simulink model "playground"  (R2024a)
settings: Solver=ode45  StartTime=0.0  StopTime=10.0  FixedStep=0.001  RelTol=1e-3
values from neighbouring files (symbols this model uses):
  a_r = 1.14 * 10^(-7)    (= 1.14e-07)    [start.m]    (also in startEnglPaper.m = 0.033; startReduced.m)
  a_rS = b    (= 0.033)    [startEnglPaper.m]
  A_x = 0.25    [playgrounMat.m]    (also in start.m; startEnglPaper.m; startReduced.m)
  A_y = 0.25    [playgrounMat.m]    (also in start.m; startEnglPaper.m; startReduced.m)
  A_z = 0.25    [playgrounMat.m]    (also in start.m; startEnglPaper.m; startReduced.m)
  b = 1.14 * 10^(-7)    (= 1.14e-07)    [start.m]    (also in startEnglPaper.m = 0.033; startReduced.m)
  g = 9.81    [playgrounMat.m]    (also in start.m; startEnglPaper.m; startReduced.m)
  gamma_d = pi/3    (= 1.0471975512)    [start.m]    (also in startReduced.m)
  I_r = 5.38 * 10 ^ (-5)    (= 5.38e-05)    [start.m]    (also in startEnglPaper.m = 3.38e-05; startReduced.m)
  I_x = 0.0151    [start.m]    (also in startEnglPaper.m = 0.004856; startReduced.m)
  I_y = 0.253    [start.m]    (also in startEnglPaper.m = 0.004856; startReduced.m)
  I_z = 0.0151    [start.m]    (also in startEnglPaper.m = 0.008801; startReduced.m)
  IrS = 5.38 * 10^(-5)    (= 5.38e-05)    [startEnglPaper.m]
  IxS = 0.0151    [startEnglPaper.m]
  IyS = IxS    (= 0.0151)    [startEnglPaper.m]
  IzS = 0.0253    [startEnglPaper.m]
  k = 1.045 * 10^(-11)    (= 1.045e-11)    [start.m]    (also in startEnglPaper.m = 2.98e-06; startReduced.m)
  K_gamma_D1 = K(1)    [playgrounMat.m]
  K_gamma_I1 = K(3)    [playgrounMat.m]
  K_gamma_P1 = K(2)    [playgrounMat.m]
  K_phi_D1 = 0.047    [startEnglPaper.m]
  K_phi_D11 = 0.093    [startEnglPaper.m]
  K_phi_D2 = 9.6    [startEnglPaper.m]
  K_phi_D22 = 19.2    [startEnglPaper.m]
  K_phi_DS = 0.14    [startEnglPaper.m]
  K_phi_I11 = 1.27    [startEnglPaper.m]
  K_phi_I22 = 262.144    [startEnglPaper.m]
  K_phi_P1 = 0.11    [startEnglPaper.m]
  K_phi_P11 = 0.5966    [startEnglPaper.m]
  K_phi_P2 = 23.04    [startEnglPaper.m]
  K_phi_P22 = 122.88    [startEnglPaper.m]
  K_phi_PS = 0.35    [startEnglPaper.m]
  K_psi_D = 40    [start.m]    (also in startEnglPaper.m = 9.6; startReduced.m)
  K_psi_D1 = 0.0844    [startEnglPaper.m]
  K_psi_D2 = 9.6    [startEnglPaper.m]
  K_psi_D22 = 19.2    [startEnglPaper.m]
  K_psi_DS = 0.24    [startEnglPaper.m]
  K_psi_I22 = 262.144    [startEnglPaper.m]
  K_psi_P = 143    [start.m]    (also in startEnglPaper.m = 23.04; startReduced.m)
  K_psi_P1 = 0.202    [startEnglPaper.m]
  K_psi_P2 = 23.04    [startEnglPaper.m]
  K_psi_P22 = 122.88    [startEnglPaper.m]
  K_psi_PS = 0.58    [startEnglPaper.m]
  K_theta_D = 58    [start.m]    (also in startEnglPaper.m = 9.6; startReduced.m)
  K_theta_D1 = 0.047    [startEnglPaper.m]
  K_theta_D2 = 9.6    [startEnglPaper.m]
  K_theta_D22 = 19.2    [startEnglPaper.m]
  K_theta_DS = 0.14    [startEnglPaper.m]
  K_theta_I22 = 262.144    [startEnglPaper.m]
  K_theta_P = 141    [start.m]    (also in startEnglPaper.m = 23.04; startReduced.m)
  K_theta_P1 = 0.11    [startEnglPaper.m]
  K_theta_P2 = 23.04    [startEnglPaper.m]
  K_theta_P22 = 122.88    [startEnglPaper.m]
  K_theta_PS = 0.35    [startEnglPaper.m]
  K_y_D = 13.58    [start.m]    (also in startReduced.m)
  K_y_P = 33.18    [start.m]    (also in startReduced.m)
  K_z_D1 = 4.42    [startEnglPaper.m]
  K_z_D2 = 4.42/m + A_z/m    (= 9.60905349794)    [startEnglPaper.m]
  K_z_DS = 13.58    [startEnglPaper.m]
  K_z_P1 = 11.2    [startEnglPaper.m]
  K_z_P2 = 11.2/m + A_z/m    (= 23.5596707819)    [startEnglPaper.m]
  K_z_PS = 33.18    [startEnglPaper.m]
  kl = 3 * 10^(-6)    (= 3e-06)    [startEnglPaper.m]
  l = 0.225    [start.m]    (also in startEnglPaper.m; startReduced.m)
  m = 1.44    [playgrounMat.m]    (also in start.m; startEnglPaper.m = 0.486; startReduced.m)
  m_s = [1/4 0 -1/(2*l) -1/(4*a_r); 1/4 -1/(2*l) 0 1/(4*a_r); 1/4 0 1/(2*l) -1/(4*a_r); 1/4 1/(2*l) 0 1/(4*a_r)]    [start.m]    (also in startReduced.m)
  mS = 1.44    [startEnglPaper.m]
  phi_d = 0.2    [startEnglPaper.m]
  phi_DesS = 0.2    [startEnglPaper.m]
  phi_init = 0    [startEnglPaper.m]
  phi_iS = 0;   deg2rad(10)    [startEnglPaper.m]
  psi_d = pi/5    (= 0.628318530718)    [start.m]    (also in startEnglPaper.m = 0.15; startReduced.m)
  psi_DesS = 0.15    [startEnglPaper.m]
  psi_init = 0    [startEnglPaper.m]
  psi_iS = 0    [startEnglPaper.m]
  theta_d = pi/4    (= 0.785398163397)    [start.m]    (also in startEnglPaper.m = 0.3; startReduced.m)
  theta_DesS = -0.1 * -3    (= 0.3)    [startEnglPaper.m]
  theta_init = 0    [startEnglPaper.m]
  theta_iS = 0    [startEnglPaper.m]
  x_init = 0    [startEnglPaper.m]
  x_iS = 0    [startEnglPaper.m]
  y_init = 0    [startEnglPaper.m]
  y_iS = 0    [startEnglPaper.m]
  z_d = 0.05 * 0    (= 0)    [startEnglPaper.m]
  z_DesS = 0.1    [startEnglPaper.m]
  z_init = 0    [startEnglPaper.m]
  z_iS = 0.0    (= 0)    [startEnglPaper.m]
undefined symbols (not defined in the file or in its folder): m_s_my
libraries: slpidlib x14
(part 2 of 4)

== system playground/ST_constants_useIX/OMEGA_2_TAU ==
  w1 : Inport
  w2 : Inport  Port=2
  w3 : Inport  Port=3
  w4 : Inport  Port=4
  Constant : Constant  Value=kl*l
  Constant1 : Constant  Value=kl*l
  Constant11 : Constant  Value=kl
  Constant7 : Constant  Value=a_rS
  Current z : Display
  Current z1 : Display
  Gyroscope : MATLAB Function  TreatAsAtomicUnit=on
  MATLAB Function : MATLAB Function  TreatAsAtomicUnit=on
  MATLAB Function1 : MATLAB Function  TreatAsAtomicUnit=on
  MATLAB Function2 : MATLAB Function  TreatAsAtomicUnit=on
  MATLAB Function3 : MATLAB Function  TreatAsAtomicUnit=on
  wR : Outport
  T_w : Outport  Port=2
  tau_phiW : Outport  Port=3
  tau_thetaW : Outport  Port=4
  tau_psiW : Outport  Port=5
  wires:
  w1/1 -> Gyroscope/1(w_1), MATLAB Function3/1(w1), MATLAB Function2/1(w1), MATLAB Function/1(w1)
  w2/1 -> Gyroscope/2(w_2), MATLAB Function3/2(w2), MATLAB Function1/1(w2), MATLAB Function/2(w2)
  w3/1 -> Gyroscope/3(w_3), MATLAB Function3/3(w3), MATLAB Function2/2(w3), MATLAB Function/3(w3)
  w4/1 -> Gyroscope/4(w_4), MATLAB Function1/2(w4), MATLAB Function/4(w4), MATLAB Function3/4(w4)
  Constant7/1 -> MATLAB Function3/5(b)
  Constant1/1 -> MATLAB Function2/3(kl)
  Constant/1 -> MATLAB Function1/3(kl)
  Constant11/1 -> MATLAB Function/5(k)
  MATLAB Function/1(T) -> Current z/1, T_w/1
  MATLAB Function1/1(tau_phi) -> Current z1/1, tau_phiW/1
  MATLAB Function2/1(tau_theta) -> tau_thetaW/1
  MATLAB Function3/1(tau_psi) -> tau_psiW/1
  Gyroscope/1(w_Gamma) -> wR/1

== system playground/ST_constants_useIX/Omega SAT ==
  w1 : Inport
  w2 : Inport  Port=2
  w3 : Inport  Port=3
  w4 : Inport  Port=4
  Current z{1..4} (4 alike) : Display
  Gain{1..4} (4 alike) : Gain  Gain=2*pi/60
  Manual Switch1 : ManualSwitch
  Manual Switch3 : ManualSwitch
  Manual Switch4 : ManualSwitch
  Manual Switch5 : ManualSwitch  CurrentSetting=0
  Sat w1 : Saturate  UpperLimit=13000  LowerLimit=1000
  Sat w2 : Saturate  UpperLimit=12500  LowerLimit=1000
  Sat w3 : Saturate  UpperLimit=12500  LowerLimit=1000
  Sat w4 : Saturate  UpperLimit=11500  LowerLimit=1000
  оборотов/мин{1..4} (4 alike) : Gain  Gain=60/(2*pi)
  w1S : Outport
  w2S : Outport  Port=2
  w3S : Outport  Port=3
  w4S : Outport  Port=4
  wires:
  w1/1 -> оборотов/мин1/1
  Gain3/1 -> Current z1/1, w3S/1  "рад/сек"
  Gain1/1 -> Current z3/1, w1S/1  "рад/сек"
  Gain2/1 -> Current z2/1, w2S/1  "рад/сек"
  Gain4/1 -> Current z4/1, w4S/1  "рад/сек"
  оборотов/мин1/1 -> Sat w1/1, Manual Switch1/1  "w1"
  Sat w1/1 -> Manual Switch1/2
  Manual Switch1/1 -> Gain1/1
  оборотов/мин2/1 -> Manual Switch3/1, Sat w2/1  "w2"
  w2/1 -> оборотов/мин2/1
  Sat w2/1 -> Manual Switch3/2
  Manual Switch3/1 -> Gain2/1
  оборотов/мин3/1 -> Sat w3/1, Manual Switch4/1  "w3"
  w3/1 -> оборотов/мин3/1
  Sat w3/1 -> Manual Switch4/2
  Manual Switch4/1 -> Gain3/1
  оборотов/мин4/1 -> Sat w4/1, Manual Switch5/1  "w4"
  w4/1 -> оборотов/мин4/1
  Sat w4/1 -> Manual Switch5/2
  Manual Switch5/1 -> Gain4/1

== system playground/ST_constants_useIX/TAU_2_OMEGA ==
  T : Inport
  tau_phi : Inport  Port=2
  tau_theta : Inport  Port=3
  tau_psi : Inport  Port=4
  Constant11 : Constant  Value=kl
  Constant12 : Constant  Value=l
  Constant7 : Constant  Value=a_rS
  Current z{,1..7} (8 alike) : Display
  MATLAB Function1 : MATLAB Function  TreatAsAtomicUnit=on
  Scope : Scope
  Sqrt{1..4} (4 alike) : Sqrt
  w1 : Outport
  w2 : Outport  Port=2
  w3 : Outport  Port=3
  w4 : Outport  Port=4
  wires:
  Constant11/1 -> MATLAB Function1/5(k)
  Constant12/1 -> MATLAB Function1/6(l)
  Constant7/1 -> MATLAB Function1/7(b)
  T/1 -> Current z4/1, MATLAB Function1/1(T)
  tau_phi/1 -> Current z5/1, MATLAB Function1/2(tau_phi)
  tau_theta/1 -> MATLAB Function1/3(tau_theta)
  tau_psi/1 -> Scope/1, Current z6/1, MATLAB Function1/4(tau_psi)
  Sqrt1/1 -> Current z/1, w1/1  "рад/сек"
  Sqrt2/1 -> Current z3/1, w2/1  "рад/сек"
  Sqrt3/1 -> Current z2/1, w3/1  "рад/сек"
  Sqrt4/1 -> Current z1/1, w4/1  "рад/сек"
  MATLAB Function1/1(omega_1) -> Sqrt1/1
  MATLAB Function1/2(omega_2) -> Current z7/1, Sqrt2/1
  MATLAB Function1/3(omega_3) -> Sqrt3/1
  MATLAB Function1/4(omega_4) -> Sqrt4/1

== system playground/ST_constants_useIX/XYZ POSITION ==
  T : Inport
  phi : Inport  Port=2
  theta : Inport  Port=3
  psi : Inport  Port=4
  Constant : Constant  Value=mS
  Constant1 : Constant  Value=A_x
  Constant2 : Constant  Value=A_y
  Constant3 : Constant  Value=A_z
  Integrator4 : Integrator
  XYZ : MATLAB Function  TreatAsAtomicUnit=on
  integrator1 : Integrator
  integrator2 : Integrator
  xinit : Integrator  InitialCondition=x_iS
  yinit : Integrator  InitialCondition=y_iS
  zinit : Integrator  InitialCondition=z_iS
  x : Outport
  y : Outport  Port=2
  z : Outport  Port=3
  wires:
  Constant3/1 -> XYZ/5(Az)
  Constant2/1 -> XYZ/4(Ay)
  integrator1/1 -> [dx], xinit/1
  integrator2/1 -> [dy], yinit/1
  Integrator4/1 -> [dz], zinit/1
  XYZ/2(ddy) -> integrator2/1
  XYZ/1(ddx) -> integrator1/1
  XYZ/3(ddz) -> Integrator4/1
  Constant1/1 -> XYZ/3(Ax)
  Constant/1 -> XYZ/2(m)
  T/1 -> XYZ/1(T)
  phi/1 -> XYZ/6(phi)
  theta/1 -> XYZ/7(theta)
  psi/1 -> XYZ/8(psi)
  [dx] -> XYZ/9(dx)
  [dy] -> XYZ/10(dy)
  [dz] -> XYZ/11(dz)
  xinit/1 -> x/1
  yinit/1 -> y/1
  zinit/1 -> z/1

== system playground/quad_PID_Simpl/9_form_omega ==
  tau_gamma : Inport
  tau_theta : Inport  Port=2
  tau_psi : Inport  Port=3
  omega_r : Inport  Port=4
  Constant1 : Constant  Value=I_z
  Constant10 : Constant  Value=I_r
  Constant11 : Constant  Value=I_y
  Constant12 : Constant  Value=I_x
  Constant2 : Constant  Value=I_z
  Constant3 : Constant  Value=I_r
  Constant4 : Constant  Value=I_y
  Constant5 : Constant  Value=I_x
  Constant6 : Constant  Value=I_y
  Constant7 : Constant  Value=I_z
  Constant8 : Constant  Value=I_x
  Integrator1 : Integrator
  Integrator2 : Integrator
  Integrator3 : Integrator
  omega_r1 : InportShadow  Port=4
  omega_x' : MATLAB Function  TreatAsAtomicUnit=on
  omega_y' : MATLAB Function  TreatAsAtomicUnit=on
  omega_z' : MATLAB Function  TreatAsAtomicUnit=on
  omega_x : Outport
  omega_y : Outport  Port=2
  omega_z : Outport  Port=3
  wires:
  Constant11/1 -> omega_y'/3(I_y)  "I_y"
  Constant12/1 -> omega_y'/2(I_x)  "I_x"
  Constant7/1 -> omega_y'/1(I_z)  "I_y"
  Constant3/1 -> omega_z'/4(I_r)  "I_r"
  Constant2/1 -> omega_z'/3(I_z)  "I_y"
  Constant5/1 -> omega_z'/2(I_x)  "I_x"
  Constant4/1 -> omega_z'/1(I_y)  "I_y"
  omega_r1/1 -> omega_x'/7(omega_r)  "omega_r"
  Constant1/1 -> omega_x'/3(I_z)  "I_y"
  omega_r/1 -> omega_z'/7(omega_r)  "omega_r"
  tau_theta/1 -> omega_z'/8(tau_theta)  "tau_theta"
  tau_psi/1 -> omega_y'/6(tau_psi)  "tau_psi"
  Integrator1/1 -> omega_y/1, omega_x'/5(omega_y), omega_z'/5(omega_y)  "omega_y"
  Integrator2/1 -> omega_z/1, omega_y'/5(omega_z), omega_x'/6(omega_z)  "omega_z"
  omega_z'/1(domega_z) -> Integrator2/1  "(omega_z)'"
  omega_y'/1(domega_y) -> Integrator1/1  "(omega_y)'"
  tau_gamma/1 -> omega_x'/8(tau_gamma)  "tau_gamma"
  Constant10/1 -> omega_x'/4(I_r)  "I_r"
  Constant8/1 -> omega_x'/2(I_x)  "I_x"
  Integrator3/1 -> omega_x/1, omega_y'/4(omega_x), omega_z'/6(omega_x)  "omega_x"
  Constant6/1 -> omega_x'/1(I_y)  "I_y"
  omega_x'/1(domega_x) -> Integrator3/1  "(omega_x)'"

== system playground/quad_PID_Simpl/Angle_moving ==
  omega_x : Inport
  omega_y : Inport  Port=2
  omega_z : Inport  Port=3
  Integrator6 : Integrator
  Integrator7 : Integrator
  Integrator8 : Integrator
  MFgamma : MATLAB Function  TreatAsAtomicUnit=on
  MFpsi : MATLAB Function  TreatAsAtomicUnit=on
  MFtheta : MATLAB Function  TreatAsAtomicUnit=on
  omega_y1 : InportShadow  Port=2
  omega_y2 : InportShadow  Port=2
  omega_z1 : InportShadow  Port=3
  omega_z2 : InportShadow  Port=3
  gamma : Outport
  theta : Outport  Port=2
  psi : Outport  Port=3
  (gamma)' : Outport  Port=4
  (theta)' : Outport  Port=5
  (psi)' : Outport  Port=6
  wires:
  omega_z1/1 -> MFtheta/2(omega_z)  "omega_z"
  omega_y1/1 -> MFtheta/1(omega_y)  "omega_y"
  omega_z2/1 -> MFpsi/2(omega_z)  "omega_z"
  omega_y2/1 -> MFpsi/1(omega_y)  "omega_y"
  omega_z/1 -> MFgamma/3(omega_z)  "omega_z"
  omega_y/1 -> MFgamma/2(omega_y)  "omega_y"
  omega_x/1 -> MFgamma/1(omega_x)  "omega_x"
  MFpsi/1(d_psi) -> (psi)'/1, Integrator8/1  "(psi)'"
  MFgamma/1(d_gamma) -> (gamma)'/1, Integrator6/1  "(gamma)'"
  Integrator7/1 -> theta/1, MFpsi/4(theta), MFgamma/5(theta)  "theta"
  Integrator6/1 -> gamma/1, MFgamma/4(gamma), MFtheta/3(gamma), MFpsi/3(gamma)  "gamma"
  Integrator8/1 -> psi/1  "psi"
  MFtheta/1(d_theta) -> (theta)'/1, Integrator7/1  "(theta)'"

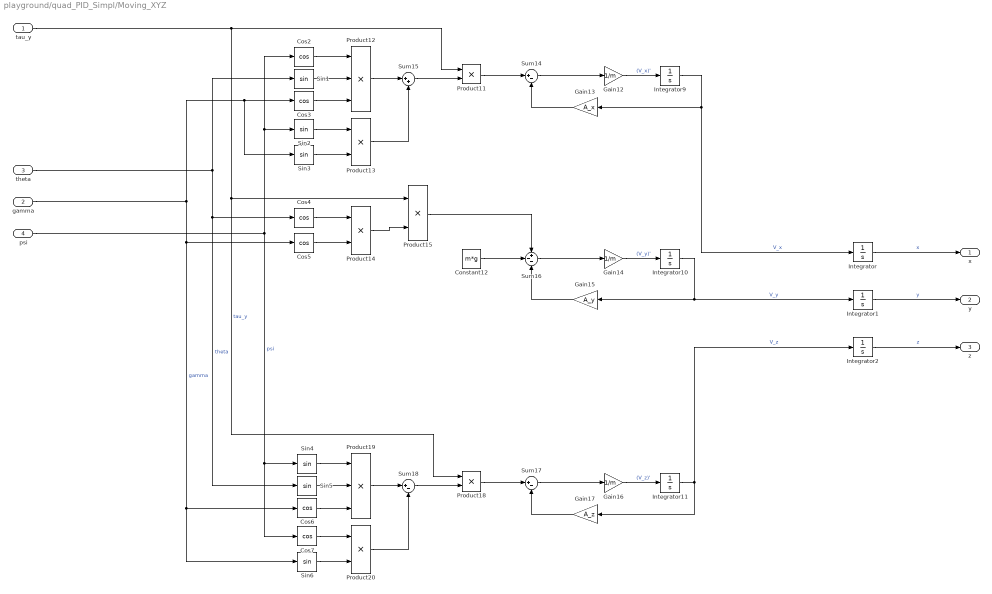
== system playground/quad_PID_Simpl/Moving_XYZ ==
  tau_y : Inport
  gamma : Inport  Port=2
  theta : Inport  Port=3
  psi : Inport  Port=4
  Constant12 : Constant  Value=m*g
  Cos{2..7} (6 alike) : Trigonometry  Operator=cos
  Gain12 : Gain  Gain=1/m
  Gain13 : Gain  Gain=A_x
  Gain14 : Gain  Gain=1/m
  Gain15 : Gain  Gain=A_y
  Gain16 : Gain  Gain=1/m
  Gain17 : Gain  Gain=A_z
  Integrator{,1..2,9..11} (6 alike) : Integrator
  Product{11,13..15,18,20} (6 alike) : Product
  Product12 : Product  Inputs=3
  Product19 : Product  Inputs=3
  Sin{1..6} (6 alike) : Trigonometry
  Sum14 : Sum  Inputs=|+-
  Sum15 : Sum  Inputs=|++
  Sum16 : Sum  Inputs=+--
  Sum17 : Sum  Inputs=|+-
  Sum18 : Sum  Inputs=|+-
  x : Outport
  y : Outport  Port=2
  z : Outport  Port=3
  wires:
  Cos4/1 -> Product14/1
  Product15/1 -> Sum16/1
  psi/1 -> Cos7/1, Sin4/1, Cos2/1, Sin2/1  "psi"
  Cos5/1 -> Product14/2
  Product11/1 -> Sum14/1
  Sin4/1 -> Product19/1
  Sin6/1 -> Product20/2
  Integrator11/1 -> Gain17/1, Integrator2/1  "V_z"
  Cos3/1 -> Product12/3
  Gain12/1 -> Integrator9/1  "(V_x)'"
  Gain16/1 -> Integrator11/1  "(V_z)'"
  Cos2/1 -> Product12/1
  tau_y/1 -> Product18/1, Product15/1, Product11/1  "tau_y"
  Product14/1 -> Product15/2
  gamma/1 -> Sin6/1, Cos6/1, Cos5/1, Sin3/1, Cos3/1  "gamma"
  theta/1 -> Sin5/1, Cos4/1, Sin1/1  "theta"
  Integrator9/1 -> Integrator/1, Gain13/1  "V_x"
  Product20/1 -> Sum18/2
  Product19/1 -> Sum18/1
  Gain14/1 -> Integrator10/1  "(V_y)'"
  Constant12/1 -> Sum16/2
  Cos7/1 -> Product20/1
  Gain17/1 -> Sum17/2
  Sin3/1 -> Product13/2
  Gain15/1 -> Sum16/3
  Sum16/1 -> Gain14/1
  Integrator10/1 -> Integrator1/1, Gain15/1  "V_y"
  Product12/1 -> Sum15/1
  Sin1/1 -> Product12/2
  Sum15/1 -> Product11/2
  Product13/1 -> Sum15/2
  Sum14/1 -> Gain12/1
  Product18/1 -> Sum17/1
  Sin2/1 -> Product13/1
  Gain13/1 -> Sum14/2
  Sum18/1 -> Product18/2
  Sum17/1 -> Gain16/1
  Cos6/1 -> Product19/3
  Sin5/1 -> Product19/2
  Integrator/1 -> x/1  "x"
  Integrator1/1 -> y/1  "y"
  Integrator2/1 -> z/1  "z"

== system playground/quad_PID_Simpl/PD regulator draft ==
  gamma : Inport
  theta : Inport  Port=2
  y : Inport  Port=3
  Constant : Constant  Value=g
  Constant1 : Constant  Value=K_y_D
  Constant4 : Constant  Value=K_y_P
  Constant7 : Constant  Value=m
  Derivative : Derivative
  Derivative1 : Derivative
  Product : Product
  Product1 : Product
  Product4 : Product
  Sum : Sum  Inputs=+++
  Sum1 : Sum  Inputs=|+-
  Sum2 : Sum  Inputs=|+-
  m/cos(y)*(cos(theta)) : MATLAB Function  TreatAsAtomicUnit=on
  target : Constant  Value=z_d
  target1 : Constant  Value=z_d
  tau_y : Outport
  wires:
  m/cos(y)*(cos(theta))/1(c) -> Product4/2
  Constant7/1 -> m/cos(y)*(cos(theta))/1(m)
  Product/1 -> Sum/1
  Constant1/1 -> Product/1
  Product1/1 -> Sum/3
  Sum1/1 -> Product/2
  Constant4/1 -> Product1/1
  target/1 -> Derivative/1
  y/1 -> Sum2/2, Derivative1/1  "y"
  Derivative1/1 -> Sum1/2
  Constant/1 -> Sum/2
  Derivative/1 -> Sum1/1
  target1/1 -> Sum2/1
  Sum2/1 -> Product1/2
  theta/1 -> m/cos(y)*(cos(theta))/3(theta)  "theta"
  gamma/1 -> m/cos(y)*(cos(theta))/2(gamma)  "gamma"
  Sum/1 -> Product4/1
  Product4/1 -> tau_y/1  "tau_y"

== system playground/quad_PID_Simpl/PD regulator gamma1 ==
  gamma : Inport
  (gamma)' : Inport  Port=2
  Constant : Constant  Value=I_x/I_x
  Constant1 : Constant  Value=K_gamma_D1
  Constant2 : Constant  Value=gamma_d
  Constant3 : Constant  Value=K_gamma_I1
  Constant4 : Constant  Value=K_gamma_P1
  Constant5 : Constant  Value=gamma_d
  Derivative : Derivative
  Integrator : Integrator
  PID Controller : slpidlib/PID Controller  Controller=PID  Form=Parallel  TimeDomain=Continuous-time  UseExternalTs=off  SampleTime=-1  IntegratorMethod=Forward Euler  FilterMethod=Forward Euler  ControllerParametersSource=internal  P=K_gamma_P1  I=K_gamma_I1  UseKiTs=off  D=K_gamma_D1  UseExternalDerivativeSource=off  N=100  UseFilter=on  TunerSelectOption=Transfer Function Based (PID Tuner App)  InitialConditionSource=internal  InitialConditionForIntegrator=0  InitialConditionForFilter=0  DifferentiatorICPrevScaledInput=0  ExternalReset=none  TrackingMode=off  Kt=1  LimitOutput=off  SatLimitsSource=internal  UpperSaturationLimit=inf  LowerSaturationLimit=-inf  LinearizeAsGain=on  AntiWindupMode=none  Kb=1  LimitIntegrator=off  UpperIntegratorSaturationLimit=inf  LowerIntegratorSaturationLimit=-inf  POutMin=[]  POutMax=[]  IOutMin=[]  IOutMax=[]  DOutMin=[]  DOutMax=[]  NOutMin=[]  NOutMax=[]  SumOutMin=[]  SumOutMax=[]  SaturationOutMin=[]  SaturationOutMax=[]  PParamMin=[]  PParamMax=[]  IParamMin=[]  IParamMax=[]  DParamMin=[]  DParamMax=[]  NParamMin=[]  NParamMax=[]  KbParamMin=[]  KbParamMax=[]  KtParamMin=[]  KtParamMax=[]  KbOutMin=[]  KbOutMax=[]  KtOutMin=[]  KtOutMax=[]  IntegratorOutMin=[]  IntegratorOutMax=[]  FilterOutMin=[]  FilterOutMax=[]  SumI1OutMin=[]  SumI1OutMax=[]  SumI2OutMin=[]  SumI2OutMax=[]  SumI3OutMin=[]  SumI3OutMax=[]  SumI4OutMin=[]  SumI4OutMax=[]  SumDOutMin=[]  SumDOutMax=[]  DifferentiatorOutMin=[]  DifferentiatorOutMax=[]  FilterDiffOutCoefMin=[]  FilterDiffOutCoefMax=[]  ReciprocalOutMin=[]  ReciprocalOutMax=[]  SumDenOutMin=[]  SumDenOutMax=[]  SumNumOutMin=[]  SumNumOutMax=[]  DivideOutMin=[]  DivideOutMax=[]  UdiffTsProdOutMin=[]  UdiffTsProdOutMax=[]  NTsProdOutMin=[]  NTsProdOutMax=[]  UintegralTsProdOutMin=[]  UintegralTsProdOutMax=[]  UngainTsProdOutMin=[]  UngainTsProdOutMax=[]  ClampingZeroOutDataTypeStr=Inherit: Inherit via back propagation  ClampingZeroOutMin=[]  ClampingZeroOutMax=[]  FilterDenConstantOutDataTypeStr=Inherit: Inherit via back propagation  FilterDenConstantOutMin=[]  FilterDenConstantOutMax=[]  PCopyOutDataTypeStr=Inherit: Inherit via back propagation  PCopyOutMin=[]  PCopyOutMax=[]  NCopyOutDataTypeStr=Inherit: Inherit via back propagation  NCopyOutMin=[]  NCopyOutMax=[]  IntegratorContinuousStateAttributes=''  IntegratorStateMustResolveToSignalObject=off  IntegratorRTWStateStorageClass=Auto  FilterContinuousStateAttributes=''  FilterStateMustResolveToSignalObject=off  FilterRTWStateStorageClass=Auto  ParallelPVariant=InternalParameters  IdealPVariant=Disabled  IVariant=InternalParameters  DVariant=InternalParameters  IntegratorVariant=Continuous  SatVariant=Disabled  AWVariant=Passthrough  PCopyVariant=Disabled  TRVariant=Disabled  FdbkBlocksVariant=Forward  IdealPFdbkVariant=Disabled  SatFdbkVariant=Disabled  DerivativeFilterVariant=ContFilter  NVariant=InternalParameters  NCopyVariant=Disabled  FilterICVariant=InternalICsFilter  IntegratorICVariant=InternalICs  ExternalResetVariant=Disabled  TRSumVariant=Passthrough  SumFdbkVariant=Disabled  SumVariant=Sum_PID  TsampFilterVariant=InternalTs  TsampNgainVariant=Passthrough  TsampIntegralVariant=Disabled_SignalSpec  ExternalSaturationOutDataTypeStr=Inherit: Same as second input  DerivativeSourceVariant=ErrorSignal
  Product{,1..3} (4 alike) : Product
  Sum : Sum  Inputs=+++|
  Sum1 : Sum  Inputs=|+-
  Sum2 : Sum  Inputs=|+-
  tau_gamma : Outport
  wires:
  Product/1 -> Sum/1
  Constant1/1 -> Product/1
  Product1/1 -> Sum/2
  Sum1/1 -> Product/2
  Constant4/1 -> Product1/1
  gamma/1 -> Sum2/2
  Constant5/1 -> Sum2/1
  Derivative/1 -> Sum1/1
  Constant2/1 -> Derivative/1
  (gamma)'/1 -> Sum1/2
  Constant/1 -> Product2/2
  Integrator/1 -> Product3/1
  Constant3/1 -> Product3/2
  Product3/1 -> Sum/3
  Sum/1 -> tau_gamma/1
  Sum2/1 -> Integrator/1, PID Controller/1, Product1/2

== system playground/quad_PID_Simpl/PD regulator psi ==
  psi : Inport
  (psi)' : Inport  Port=2
  Constant : Constant  Value=I_y/I_y
  Constant1 : Constant  Value=K_psi_D
  Constant2 : Constant  Value=psi_d
  Constant4 : Constant  Value=K_psi_P
  Constant5 : Constant  Value=psi_d
  Derivative : Derivative
  Product : Product
  Product1 : Product
  Product2 : Product
  Sum : Sum  Inputs=++|
  Sum1 : Sum  Inputs=|+-
  Sum2 : Sum  Inputs=|+-
  tau_psi : Outport
  wires:
  Product/1 -> Sum/1
  Constant1/1 -> Product/1
  Product1/1 -> Sum/2
  Sum1/1 -> Product/2
  Constant4/1 -> Product1/1
  psi/1 -> Sum2/2
  Constant5/1 -> Sum2/1
  Derivative/1 -> Sum1/1
  Constant2/1 -> Derivative/1
  (psi)'/1 -> Sum1/2
  Sum2/1 -> Product1/2
  Product2/1 -> tau_psi/1  "tau_psi"
  Constant/1 -> Product2/2
  Sum/1 -> Product2/1

== system playground/quad_PID_Simpl/PD regulator theta ==
  theta : Inport
  (theta)' : Inport  Port=2
  Constant : Constant  Value=I_z/I_z
  Constant1 : Constant  Value=K_theta_D
  Constant2 : Constant  Value=theta_d
  Constant4 : Constant  Value=K_theta_P
  Constant5 : Constant  Value=theta_d
  Derivative : Derivative
  Product : Product
  Product1 : Product
  Product2 : Product
  Sum : Sum  Inputs=++|
  Sum1 : Sum  Inputs=|+-
  Sum2 : Sum  Inputs=|+-
  tau_theta : Outport
  wires:
  Product/1 -> Sum/1
  Constant1/1 -> Product/1
  Product1/1 -> Sum/2
  Sum1/1 -> Product/2
  Constant4/1 -> Product1/1
  theta/1 -> Sum2/2
  Constant5/1 -> Sum2/1
  Derivative/1 -> Sum1/1
  Constant2/1 -> Derivative/1
  (theta)'/1 -> Sum1/2
  Sum2/1 -> Product1/2
  Product2/1 -> tau_theta/1  "tau_theta"
  Constant/1 -> Product2/2
  Sum/1 -> Product2/1

== system playground/quad_PID_Simpl/Subsystem3 ==
  omega_1 : Inport
  omega_2 : Inport  Port=2
  omega_3 : Inport  Port=3
  omega_4 : Inport  Port=4
  Gain1 : Gain  Gain=l*k
  Gain2 : Gain  Gain=l*k
  Gain3 : Gain  Gain=b
  Gain4 : Gain  Gain=k
  Math Function{,1..5} (6 alike) : Math  Operator=square  SignedPower=on
  Mux : Mux
  Mux1 : Mux
  Sum of Elements : Sum  Inputs=+
  Sum of Elements1 : Sum  Inputs=+
  Sum1 : Sum  Inputs=|-+
  Sum2 : Sum  Inputs=|-+
  tau_gamma : Outport
  tau_theta : Outport  Port=2
  tau_psi : Outport  Port=3
  tau_y : Outport  Port=4
  wires:
  Gain1/1 -> tau_theta/1
  Sum2/1 -> Gain1/1
  Sum1/1 -> Gain2/1
  Gain2/1 -> tau_gamma/1
  Math Function/1 -> Sum1/1
  Math Function1/1 -> Sum1/2
  Math Function2/1 -> Sum2/1
  Math Function3/1 -> Sum2/2
  Mux/1 -> Math Function4/1
  Math Function4/1 -> Gain3/1
  Gain3/1 -> Sum of Elements/1
  Sum of Elements/1 -> tau_psi/1
  Sum of Elements1/1 -> tau_y/1
  Gain4/1 -> Sum of Elements1/1
  Math Function5/1 -> Gain4/1
  Mux1/1 -> Math Function5/1
  omega_2/1 -> Mux1/2, Mux/2, Math Function/1
  omega_3/1 -> Math Function3/1, Mux1/3, Mux/3
  omega_1/1 -> Math Function2/1, Mux1/1, Mux/1
  omega_4/1 -> Mux1/4, Mux/4, Math Function1/1

== system playground/quad_PID_Simpl/Subsystem4 ==
  omega_1 : Inport
  omega_2 : Inport  Port=2
  omega_3 : Inport  Port=3
  omega_4 : Inport  Port=4
  Gain1 : Gain  Gain=l*k
  Gain2 : Gain  Gain=l*k
  Gain3 : Gain  Gain=b
  Gain4 : Gain  Gain=k
  Math Function{,1..5} (6 alike) : Math  Operator=square  SignedPower=on
  Mux : Mux
  Mux1 : Mux
  Sum of Elements : Sum  Inputs=+
  Sum of Elements1 : Sum  Inputs=+
  Sum1 : Sum  Inputs=|-+
  Sum2 : Sum  Inputs=|-+
  tau_gamma : Outport
  tau_theta : Outport  Port=2
  tau_psi : Outport  Port=3
  tau_y : Outport  Port=4
  wires:
  Gain1/1 -> tau_theta/1
  Sum2/1 -> Gain1/1
  Sum1/1 -> Gain2/1
  Gain2/1 -> tau_gamma/1
  Math Function/1 -> Sum1/1
  Math Function1/1 -> Sum1/2
  Math Function2/1 -> Sum2/1
  Math Function3/1 -> Sum2/2
  Mux/1 -> Math Function4/1
  Math Function4/1 -> Gain3/1
  Gain3/1 -> Sum of Elements/1
  Sum of Elements/1 -> tau_psi/1
  Sum of Elements1/1 -> tau_y/1
  Gain4/1 -> Sum of Elements1/1
  Math Function5/1 -> Gain4/1
  Mux1/1 -> Math Function5/1
  omega_2/1 -> Mux1/2, Mux/2, Math Function/1
  omega_3/1 -> Math Function3/1, Mux1/3, Mux/3
  omega_1/1 -> Math Function2/1, Mux1/1, Mux/1
  omega_4/1 -> Mux1/4, Mux/4, Math Function1/1

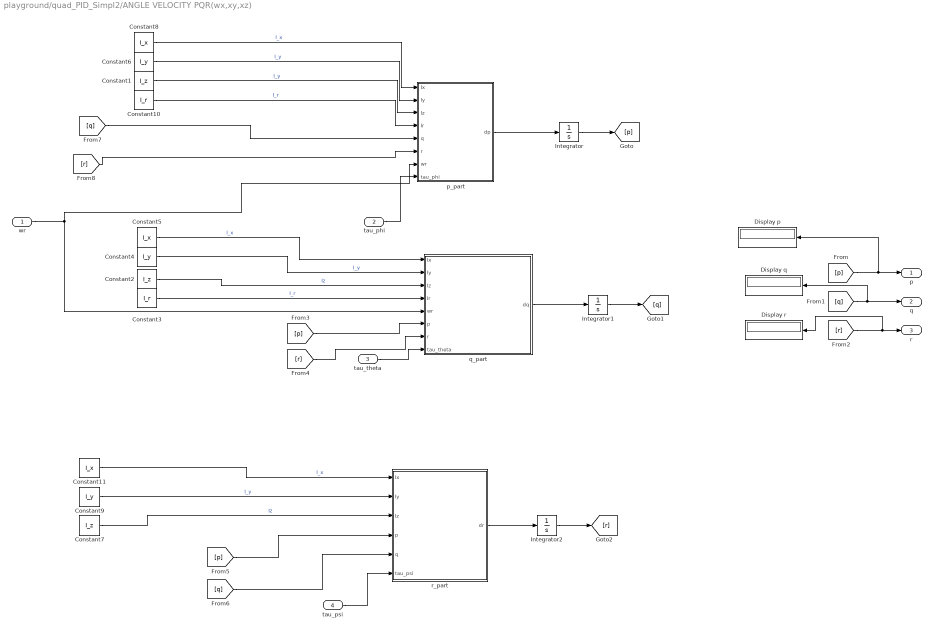
== system playground/quad_PID_Simpl2/ANGLE VELOCITY PQR(wx,xy,xz) ==
  wr : Inport
  tau_phi : Inport  Port=2
  tau_theta : Inport  Port=3
  tau_psi : Inport  Port=4
  Constant1 : Constant  Value=I_z
  Constant10 : Constant  Value=I_r
  Constant11 : Constant  Value=I_x
  Constant2 : Constant  Value=I_z
  Constant3 : Constant  Value=I_r
  Constant4 : Constant  Value=I_y
  Constant5 : Constant  Value=I_x
  Constant6 : Constant  Value=I_y
  Constant7 : Constant  Value=I_z
  Constant8 : Constant  Value=I_x
  Constant9 : Constant  Value=I_y
  Display p : Display
  Display q : Display
  Display r : Display
  Integrator : Integrator
  Integrator1 : Integrator
  Integrator2 : Integrator
  p_part : MATLAB Function  TreatAsAtomicUnit=on
  q_part : MATLAB Function  TreatAsAtomicUnit=on
  r_part : MATLAB Function  TreatAsAtomicUnit=on
  p : Outport
  q : Outport  Port=2
  r : Outport  Port=3
  wires:
  Constant8/1 -> p_part/1(Ix)  "I_x"
  Constant6/1 -> p_part/2(Iy)  "I_y"
  Constant1/1 -> p_part/3(Iz)  "I_y"
  Constant10/1 -> p_part/4(Ir)  "I_r"
  Constant5/1 -> q_part/1(Ix)  "I_x"
  Constant4/1 -> q_part/2(Iy)  "I_y"
  Constant2/1 -> q_part/3(Iz)  "Iz"
  Constant3/1 -> q_part/4(Ir)  "I_r"
  Constant11/1 -> r_part/1(Ix)  "I_x"
  Constant9/1 -> r_part/2(Iy)  "I_y"
  Constant7/1 -> r_part/3(Iz)  "Iz"
  wr/1 -> p_part/7(wr), q_part/5(wr)
  tau_psi/1 -> r_part/6(tau_psi)
  tau_phi/1 -> p_part/8(tau_phi)
  tau_theta/1 -> q_part/8(tau_theta)
  p_part/1(dp) -> Integrator/1
  q_part/1(dq) -> Integrator1/1
  r_part/1(dr) -> Integrator2/1
  Integrator1/1 -> [q]
  Integrator/1 -> [p]
  Integrator2/1 -> [r]
  [p] -> q_part/6(p)
  [r] -> q_part/7(r)
  [p] -> r_part/4(p)
  [q] -> r_part/5(q)
  [q] -> p_part/5(q)
  [r] -> p_part/6(r)
  [p] -> p/1, Display p/1
  [q] -> q/1, Display q/1
  [r] -> r/1, Display r/1

== system playground/quad_PID_Simpl2/ANGLS ==
  p : Inport
  q : Inport  Port=2
  r : Inport  Port=3
  Current z : Display
  Integrator : Integrator  InitialCondition=phi_init
  Integrator1 : Integrator  InitialCondition=theta_init
  Integrator2 : Integrator  InitialCondition=psi_init
  phi_part : MATLAB Function  TreatAsAtomicUnit=on
  psi_part : MATLAB Function  TreatAsAtomicUnit=on
  q1 : InportShadow  Port=2
  q2 : InportShadow  Port=2
  r1 : InportShadow  Port=3
  r2 : InportShadow  Port=3
  theta_part : MATLAB Function  TreatAsAtomicUnit=on
  phi : Outport
  theta : Outport  Port=2
  psi : Outport  Port=3
  dphi : Outport  Port=4
  dtheta : Outport  Port=5
  dpsi : Outport  Port=6
  wires:
  phi_part/1(d_phi) -> dphi/1, Integrator/1
  Integrator/1 -> Current z/1, [phi]
  theta_part/1(d_theta) -> dtheta/1, Integrator1/1
  Integrator1/1 -> [theta]
  psi_part/1(d_psi) -> dpsi/1, Integrator2/1
  Integrator2/1 -> [psi]
  [phi] -> phi_part/4(phi)
  [phi] -> theta_part/3(phi)
  [phi] -> psi_part/3(phi)
  [theta] -> psi_part/4(theta)
  [theta] -> phi_part/5(theta)
  p/1 -> phi_part/1(p)
  q/1 -> phi_part/2(q)
  r/1 -> phi_part/3(r)
  q1/1 -> theta_part/1(q)
  q2/1 -> psi_part/1(q)
  r1/1 -> theta_part/2(r)
  r2/1 -> psi_part/2(r)
  [psi] -> psi/1
  [theta] -> theta/1
  [phi] -> phi/1

== system playground/quad_PID_Simpl2/CONTROLLER ==
  phi : Inport
  dphi : Inport  Port=2
  theta : Inport  Port=3
  dtheta : Inport  Port=4
  psi : Inport  Port=5
  dpsi : Inport  Port=6
  z : Inport  Port=7
  Current z : Display
  Current z1 : Display
  Current z2 : Display
  PD regulator draft : Subsystem
  PD regulator gamma1 : Subsystem
  PD regulator psi : Subsystem
  PD regulator theta : Subsystem
  T : Outport
  tau_phi : Outport  Port=2
  tau_theta : Outport  Port=3
  tau_psi : Outport  Port=4
  wires:
  z/1 -> PD regulator draft/3(z)
  phi/1 -> PD regulator gamma1/1(phi), PD regulator draft/1(phi)
  theta/1 -> PD regulator draft/2(theta), PD regulator theta/1(theta)
  dtheta/1 -> PD regulator theta/2((theta)')
  dphi/1 -> PD regulator gamma1/2((phi)')
  psi/1 -> PD regulator psi/1(psi)
  dpsi/1 -> PD regulator psi/2((psi)')
  PD regulator psi/1(tau_psi) -> Current z2/1, tau_psi/1  "tau_psi"
  PD regulator theta/1(tau_theta) -> tau_theta/1  "tau_theta"
  PD regulator gamma1/1(tau_phi) -> Current z1/1, tau_phi/1  "tau_gamma"
  PD regulator draft/1(T) -> Current z/1, T/1  "tau_y"

== system playground/quad_PID_Simpl2/OMEGA_2_TAU ==
  w1 : Inport
  w2 : Inport  Port=2
  w3 : Inport  Port=3
  w4 : Inport  Port=4
  Constant : Constant  Value=kl*l
  Constant1 : Constant  Value=kl*l
  Constant11 : Constant  Value=kl
  Constant7 : Constant  Value=b
  Current z : Display
  Current z1 : Display
  Gain7 : Gain  Gain=2*pi/60
  Gyroscope : MATLAB Function  TreatAsAtomicUnit=on
  MATLAB Function : MATLAB Function  TreatAsAtomicUnit=on
  MATLAB Function1 : MATLAB Function  TreatAsAtomicUnit=on
  MATLAB Function2 : MATLAB Function  TreatAsAtomicUnit=on
  MATLAB Function3 : MATLAB Function  TreatAsAtomicUnit=on
  Manual Switch : ManualSwitch
  Scope : Scope
  Scope1 : Scope
  оборотов/мин1 : Gain  Gain=60/(2*pi)
  wR : Outport
  T_w : Outport  Port=2
  tau_phiW : Outport  Port=3
  tau_thetaW : Outport  Port=4
  tau_psiW : Outport  Port=5
  wires:
  Manual Switch/1 -> Gyroscope/1(w_1), MATLAB Function3/1(w1), MATLAB Function2/1(w1), MATLAB Function/1(w1)
  w2/1 -> Gyroscope/2(w_2), MATLAB Function3/2(w2), MATLAB Function1/1(w2), MATLAB Function/2(w2)
  w3/1 -> Gyroscope/3(w_3), MATLAB Function3/3(w3), MATLAB Function2/2(w3), MATLAB Function/3(w3)
  w4/1 -> Gyroscope/4(w_4), MATLAB Function1/2(w4), MATLAB Function/4(w4), MATLAB Function3/4(w4)
  Constant7/1 -> MATLAB Function3/5(b)
  Constant1/1 -> MATLAB Function2/3(kl)
  Constant/1 -> MATLAB Function1/3(kl)
  Constant11/1 -> MATLAB Function/5(k)
  MATLAB Function/1(T) -> Current z/1, T_w/1
  MATLAB Function1/1(tau_phi) -> Current z1/1, tau_phiW/1
  MATLAB Function2/1(tau_theta) -> tau_thetaW/1
  MATLAB Function3/1(tau_psi) -> Scope/1, tau_psiW/1
  Gyroscope/1(w_Gamma) -> wR/1
  MATLAB Function3/2(err) -> Scope1/1
  w1/1 -> Manual Switch/2, оборотов/мин1/1
  оборотов/мин1/1 -> Gain7/1  "w1"
  Gain7/1 -> Manual Switch/1

== system playground/quad_PID_Simpl2/Omega SAT ==
  w1 : Inport
  w2 : Inport  Port=2
  w3 : Inport  Port=3
  w4 : Inport  Port=4
  Current z{1..4} (4 alike) : Display
  Gain{1..4} (4 alike) : Gain  Gain=2*pi/60
  Manual Switch1 : ManualSwitch
  Manual Switch3 : ManualSwitch
  Manual Switch4 : ManualSwitch
  Manual Switch5 : ManualSwitch  CurrentSetting=0
  Sat w1 : Saturate  UpperLimit=7000  LowerLimit=1000
  Sat w2 : Saturate  UpperLimit=7200  LowerLimit=1000
  Sat w3 : Saturate  UpperLimit=6400  LowerLimit=1000
  Sat w4 : Saturate  UpperLimit=6600  LowerLimit=1000
  оборотов/мин{1..4} (4 alike) : Gain  Gain=60/(2*pi)
  w1S : Outport
  w2S : Outport  Port=2
  w3S : Outport  Port=3
  w4S : Outport  Port=4
  wires:
  w1/1 -> оборотов/мин1/1
  Gain3/1 -> Current z1/1, w3S/1  "рад/сек"
  Gain1/1 -> Current z3/1, w1S/1  "рад/сек"
  Gain2/1 -> Current z2/1, w2S/1  "рад/сек"
  Gain4/1 -> Current z4/1, w4S/1  "рад/сек"
  оборотов/мин1/1 -> Sat w1/1, Manual Switch1/1  "w1"
  Sat w1/1 -> Manual Switch1/2
  Manual Switch1/1 -> Gain1/1
  оборотов/мин2/1 -> Manual Switch3/1, Sat w2/1  "w2"
  w2/1 -> оборотов/мин2/1
  Sat w2/1 -> Manual Switch3/2
  Manual Switch3/1 -> Gain2/1
  оборотов/мин3/1 -> Sat w3/1, Manual Switch4/1  "w3"
  w3/1 -> оборотов/мин3/1
  Sat w3/1 -> Manual Switch4/2
  Manual Switch4/1 -> Gain3/1
  оборотов/мин4/1 -> Sat w4/1, Manual Switch5/1  "w4"
  w4/1 -> оборотов/мин4/1
  Sat w4/1 -> Manual Switch5/2
  Manual Switch5/1 -> Gain4/1

== system playground/quad_PID_Simpl2/TAU_2_OMEGA ==
  T : Inport
  tau_phi : Inport  Port=2
  tau_theta : Inport  Port=3
  tau_psi : Inport  Port=4
  Constant11 : Constant  Value=kl
  Constant12 : Constant  Value=l
  Constant7 : Constant  Value=b
  Current z{,1..8} (9 alike) : Display
  MATLAB Function1 : MATLAB Function  TreatAsAtomicUnit=on
  Scope : Scope
  Sqrt{1..4} (4 alike) : Sqrt
  w1 : Outport
  w2 : Outport  Port=2
  w3 : Outport  Port=3
  w4 : Outport  Port=4
  wires:
  Constant11/1 -> MATLAB Function1/5(k)
  Constant12/1 -> MATLAB Function1/6(l)
  Constant7/1 -> MATLAB Function1/7(b)
  T/1 -> Current z4/1, MATLAB Function1/1(T)
  tau_phi/1 -> MATLAB Function1/2(tau_phi), Current z5/1
  tau_theta/1 -> Current z8/1, MATLAB Function1/3(tau_theta)
  tau_psi/1 -> Scope/1, Current z6/1, MATLAB Function1/4(tau_psi)
  Sqrt1/1 -> Current z/1, w1/1  "рад/сек"
  Sqrt2/1 -> Current z3/1, w2/1  "рад/сек"
  Sqrt3/1 -> Current z2/1, w3/1  "рад/сек"
  Sqrt4/1 -> Current z1/1, w4/1  "рад/сек"
  MATLAB Function1/1(omega_1) -> Sqrt1/1
  MATLAB Function1/2(omega_2) -> Current z7/1, Sqrt2/1
  MATLAB Function1/3(omega_3) -> Sqrt3/1
  MATLAB Function1/4(omega_4) -> Sqrt4/1

== system playground/quad_PID_Simpl2/XYZ POSITION ==
  T : Inport
  phi : Inport  Port=2
  theta : Inport  Port=3
  psi : Inport  Port=4
  Constant : Constant  Value=m
  Constant1 : Constant  Value=A_x
  Constant2 : Constant  Value=A_y
  Constant3 : Constant  Value=A_z
  Integrator4 : Integrator
  XYZ : MATLAB Function  TreatAsAtomicUnit=on
  integrator1 : Integrator
  integrator2 : Integrator
  xinit : Integrator  InitialCondition=x_init
  yinit : Integrator  InitialCondition=y_init
  zinit : Integrator  InitialCondition=z_init
  x : Outport
  y : Outport  Port=2
  z : Outport  Port=3
  wires:
  Constant3/1 -> XYZ/5(Az)
  Constant2/1 -> XYZ/4(Ay)
  integrator1/1 -> [dx], xinit/1
  integrator2/1 -> [dy], yinit/1
  Integrator4/1 -> [dz], zinit/1
  XYZ/2(ddy) -> integrator2/1
  XYZ/1(ddx) -> integrator1/1
  XYZ/3(ddz) -> Integrator4/1
  Constant1/1 -> XYZ/3(Ax)
  Constant/1 -> XYZ/2(m)
  T/1 -> XYZ/1(T)
  phi/1 -> XYZ/6(phi)
  theta/1 -> XYZ/7(theta)
  psi/1 -> XYZ/8(psi)
  [dx] -> XYZ/9(dx)
  [dy] -> XYZ/10(dy)
  [dz] -> XYZ/11(dz)
  xinit/1 -> x/1
  yinit/1 -> y/1
  zinit/1 -> z/1

== system playground/CHANGE_PID/CONTROLLER/PD regulator draft ==
  phi : Inport
  theta : Inport  Port=2
  z : Inport  Port=3
  Altitude controller : slpidlib/PID Controller  Controller=PID  Form=Parallel  TimeDomain=Continuous-time  UseExternalTs=off  SampleTime=-1  IntegratorMethod=Forward Euler  FilterMethod=Forward Euler  ControllerParametersSource=internal  P=K_z_P1  I=0  UseKiTs=off  D=K_z_D1  UseExternalDerivativeSource=off  N=100  UseFilter=on  TunerSelectOption=Transfer Function Based (PID Tuner App)  InitialConditionSource=internal  InitialConditionForIntegrator=0  InitialConditionForFilter=0  DifferentiatorICPrevScaledInput=0  ExternalReset=none  TrackingMode=off  Kt=1  LimitOutput=on  SatLimitsSource=internal  UpperSaturationLimit=5  LowerSaturationLimit=-5  LinearizeAsGain=on  AntiWindupMode=none  Kb=1  LimitIntegrator=off  UpperIntegratorSaturationLimit=inf  LowerIntegratorSaturationLimit=-inf  POutMin=[]  POutMax=[]  IOutMin=[]  IOutMax=[]  DOutMin=[]  DOutMax=[]  NOutMin=[]  NOutMax=[]  SumOutMin=[]  SumOutMax=[]  SaturationOutMin=[]  SaturationOutMax=[]  PParamMin=[]  PParamMax=[]  IParamMin=[]  IParamMax=[]  DParamMin=[]  DParamMax=[]  NParamMin=[]  NParamMax=[]  KbParamMin=[]  KbParamMax=[]  KtParamMin=[]  KtParamMax=[]  KbOutMin=[]  KbOutMax=[]  KtOutMin=[]  KtOutMax=[]  IntegratorOutMin=[]  IntegratorOutMax=[]  FilterOutMin=[]  FilterOutMax=[]  SumI1OutMin=[]  SumI1OutMax=[]  SumI2OutMin=[]  SumI2OutMax=[]  SumI3OutMin=[]  SumI3OutMax=[]  SumI4OutMin=[]  SumI4OutMax=[]  SumDOutMin=[]  SumDOutMax=[]  DifferentiatorOutMin=[]  DifferentiatorOutMax=[]  FilterDiffOutCoefMin=[]  FilterDiffOutCoefMax=[]  ReciprocalOutMin=[]  ReciprocalOutMax=[]  SumDenOutMin=[]  SumDenOutMax=[]  SumNumOutMin=[]  SumNumOutMax=[]  DivideOutMin=[]  DivideOutMax=[]  UdiffTsProdOutMin=[]  UdiffTsProdOutMax=[]  NTsProdOutMin=[]  NTsProdOutMax=[]  UintegralTsProdOutMin=[]  UintegralTsProdOutMax=[]  UngainTsProdOutMin=[]  UngainTsProdOutMax=[]  ClampingZeroOutDataTypeStr=Inherit: Inherit via back propagation  ClampingZeroOutMin=[]  ClampingZeroOutMax=[]  FilterDenConstantOutDataTypeStr=Inherit: Inherit via back propagation  FilterDenConstantOutMin=[]  FilterDenConstantOutMax=[]  PCopyOutDataTypeStr=Inherit: Inherit via back propagation  PCopyOutMin=[]  PCopyOutMax=[]  NCopyOutDataTypeStr=Inherit: Inherit via back propagation  NCopyOutMin=[]  NCopyOutMax=[]  IntegratorContinuousStateAttributes=''  IntegratorStateMustResolveToSignalObject=off  IntegratorRTWStateStorageClass=Auto  FilterContinuousStateAttributes=''  FilterStateMustResolveToSignalObject=off  FilterRTWStateStorageClass=Auto  ParallelPVariant=InternalParameters  IdealPVariant=Disabled  IVariant=InternalParameters  DVariant=InternalParameters  IntegratorVariant=Continuous  SatVariant=Enabled  AWVariant=Passthrough  PCopyVariant=Disabled  TRVariant=Disabled  FdbkBlocksVariant=Forward  IdealPFdbkVariant=Disabled  SatFdbkVariant=Disabled  DerivativeFilterVariant=ContFilter  NVariant=InternalParameters  NCopyVariant=Disabled  FilterICVariant=InternalICsFilter  IntegratorICVariant=InternalICs  ExternalResetVariant=Disabled  TRSumVariant=Passthrough  SumFdbkVariant=Disabled  SumVariant=Sum_PID  TsampFilterVariant=InternalTs  TsampNgainVariant=Passthrough  TsampIntegralVariant=Disabled_SignalSpec  ExternalSaturationOutDataTypeStr=Inherit: Same as second input  DerivativeSourceVariant=ErrorSignal
  Constant : Constant  Value=g
  Constant7 : Constant  Value=m
  Derivative1 : Derivative
  Derivative2 : Derivative
  Gain : Gain  Gain=K_z_D1
  Gain1 : Gain  Gain=K_z_P1
  Product4 : Product
  Sum : Sum  Inputs=+++
  Sum1 : Sum  Inputs=|+-
  Sum2 : Sum  Inputs=|-+
  m/cos(y)*(cos(theta)) : MATLAB Function  TreatAsAtomicUnit=on
  target2 : Constant  Value=z_d
  target3 : Constant  Value=z_d
  T : Outport
  wires:
  target3/1 -> Sum2/2
  target2/1 -> Derivative2/1
  m/cos(y)*(cos(theta))/1(c) -> Product4/2
  Constant7/1 -> m/cos(y)*(cos(theta))/1(m)
  Sum1/1 -> Gain/1
  z/1 -> Derivative1/1, Sum2/1  "z"
  Derivative1/1 -> Sum1/2
  Constant/1 -> Sum/2
  Derivative2/1 -> Sum1/1
  theta/1 -> m/cos(y)*(cos(theta))/3(theta)  "theta"
  phi/1 -> m/cos(y)*(cos(theta))/2(phi)  "gamma"
  Sum/1 -> Product4/1
  Product4/1 -> T/1  "T"
  Sum2/1 -> Altitude controller/1, Gain1/1
  Altitude controller/1 -> Sum/3

== system playground/CHANGE_PID/CONTROLLER/PD regulator gamma1 ==
  phi : Inport
  (phi)' : Inport  Port=2
  Altitude controller : slpidlib/PID Controller  Controller=PID  Form=Parallel  TimeDomain=Continuous-time  UseExternalTs=off  SampleTime=-1  IntegratorMethod=Forward Euler  FilterMethod=Forward Euler  ControllerParametersSource=internal  P=K_phi_P11  I=K_phi_I11  UseKiTs=off  D=K_phi_D11  UseExternalDerivativeSource=off  N=100  UseFilter=on  TunerSelectOption=Transfer Function Based (PID Tuner App)  InitialConditionSource=internal  InitialConditionForIntegrator=0  InitialConditionForFilter=0  DifferentiatorICPrevScaledInput=0  ExternalReset=none  TrackingMode=off  Kt=1  LimitOutput=on  SatLimitsSource=internal  UpperSaturationLimit=5  LowerSaturationLimit=-5  LinearizeAsGain=on  AntiWindupMode=none  Kb=1  LimitIntegrator=off  UpperIntegratorSaturationLimit=inf  LowerIntegratorSaturationLimit=-inf  POutMin=[]  POutMax=[]  IOutMin=[]  IOutMax=[]  DOutMin=[]  DOutMax=[]  NOutMin=[]  NOutMax=[]  SumOutMin=[]  SumOutMax=[]  SaturationOutMin=[]  SaturationOutMax=[]  PParamMin=[]  PParamMax=[]  IParamMin=[]  IParamMax=[]  DParamMin=[]  DParamMax=[]  NParamMin=[]  NParamMax=[]  KbParamMin=[]  KbParamMax=[]  KtParamMin=[]  KtParamMax=[]  KbOutMin=[]  KbOutMax=[]  KtOutMin=[]  KtOutMax=[]  IntegratorOutMin=[]  IntegratorOutMax=[]  FilterOutMin=[]  FilterOutMax=[]  SumI1OutMin=[]  SumI1OutMax=[]  SumI2OutMin=[]  SumI2OutMax=[]  SumI3OutMin=[]  SumI3OutMax=[]  SumI4OutMin=[]  SumI4OutMax=[]  SumDOutMin=[]  SumDOutMax=[]  DifferentiatorOutMin=[]  DifferentiatorOutMax=[]  FilterDiffOutCoefMin=[]  FilterDiffOutCoefMax=[]  ReciprocalOutMin=[]  ReciprocalOutMax=[]  SumDenOutMin=[]  SumDenOutMax=[]  SumNumOutMin=[]  SumNumOutMax=[]  DivideOutMin=[]  DivideOutMax=[]  UdiffTsProdOutMin=[]  UdiffTsProdOutMax=[]  NTsProdOutMin=[]  NTsProdOutMax=[]  UintegralTsProdOutMin=[]  UintegralTsProdOutMax=[]  UngainTsProdOutMin=[]  UngainTsProdOutMax=[]  ClampingZeroOutDataTypeStr=Inherit: Inherit via back propagation  ClampingZeroOutMin=[]  ClampingZeroOutMax=[]  FilterDenConstantOutDataTypeStr=Inherit: Inherit via back propagation  FilterDenConstantOutMin=[]  FilterDenConstantOutMax=[]  PCopyOutDataTypeStr=Inherit: Inherit via back propagation  PCopyOutMin=[]  PCopyOutMax=[]  NCopyOutDataTypeStr=Inherit: Inherit via back propagation  NCopyOutMin=[]  NCopyOutMax=[]  IntegratorContinuousStateAttributes=''  IntegratorStateMustResolveToSignalObject=off  IntegratorRTWStateStorageClass=Auto  FilterContinuousStateAttributes=''  FilterStateMustResolveToSignalObject=off  FilterRTWStateStorageClass=Auto  ParallelPVariant=InternalParameters  IdealPVariant=Disabled  IVariant=InternalParameters  DVariant=InternalParameters  IntegratorVariant=Continuous  SatVariant=Enabled  AWVariant=Passthrough  PCopyVariant=Disabled  TRVariant=Disabled  FdbkBlocksVariant=Forward  IdealPFdbkVariant=Disabled  SatFdbkVariant=Disabled  DerivativeFilterVariant=ContFilter  NVariant=InternalParameters  NCopyVariant=Disabled  FilterICVariant=InternalICsFilter  IntegratorICVariant=InternalICs  ExternalResetVariant=Disabled  TRSumVariant=Passthrough  SumFdbkVariant=Disabled  SumVariant=Sum_PID  TsampFilterVariant=InternalTs  TsampNgainVariant=Passthrough  TsampIntegralVariant=Disabled_SignalSpec  ExternalSaturationOutDataTypeStr=Inherit: Same as second input  DerivativeSourceVariant=ErrorSignal
  Constant : Constant  Value=I_x/I_x
  Constant2 : Constant  Value=phi_d
  Constant5 : Constant  Value=phi_d
  Current x : Display
  Current x1 : Display
  Derivative : Derivative
  Gain : Gain  Gain=K_phi_D1
  Gain1 : Gain  Gain=K_phi_P1
  Product2 : Product
  Sum : Sum  Inputs=++|
  Sum1 : Sum  Inputs=|+-
  Sum2 : Sum  Inputs=|+-
  tau_phi : Outport
  wires:
  Gain1/1 -> Sum/2
  Sum2/1 -> Altitude controller/1, Gain1/1
  Gain/1 -> Sum/1
  Product2/1 -> tau_phi/1  "tau_gamma"
  Sum1/1 -> Gain/1
  phi/1 -> Sum2/2
  Constant5/1 -> Sum2/1
  Derivative/1 -> Sum1/1
  Constant2/1 -> Derivative/1
  (phi)'/1 -> Sum1/2
  Constant/1 -> Product2/2
  Sum/1 -> Current x/1
  Altitude controller/1 -> Current x1/1, Product2/1

== system playground/CHANGE_PID/CONTROLLER/PD regulator psi ==
  psi : Inport
  (psi)' : Inport  Port=2
  Altitude controller : slpidlib/PID Controller  Controller=PID  Form=Parallel  TimeDomain=Continuous-time  UseExternalTs=off  SampleTime=-1  IntegratorMethod=Forward Euler  FilterMethod=Forward Euler  ControllerParametersSource=internal  P=K_psi_P1  I=0  UseKiTs=off  D=K_psi_D1  UseExternalDerivativeSource=off  N=100  UseFilter=on  TunerSelectOption=Transfer Function Based (PID Tuner App)  InitialConditionSource=internal  InitialConditionForIntegrator=0  InitialConditionForFilter=0  DifferentiatorICPrevScaledInput=0  ExternalReset=none  TrackingMode=off  Kt=1  LimitOutput=on  SatLimitsSource=internal  UpperSaturationLimit=5  LowerSaturationLimit=-5  LinearizeAsGain=on  AntiWindupMode=none  Kb=1  LimitIntegrator=off  UpperIntegratorSaturationLimit=inf  LowerIntegratorSaturationLimit=-inf  POutMin=[]  POutMax=[]  IOutMin=[]  IOutMax=[]  DOutMin=[]  DOutMax=[]  NOutMin=[]  NOutMax=[]  SumOutMin=[]  SumOutMax=[]  SaturationOutMin=[]  SaturationOutMax=[]  PParamMin=[]  PParamMax=[]  IParamMin=[]  IParamMax=[]  DParamMin=[]  DParamMax=[]  NParamMin=[]  NParamMax=[]  KbParamMin=[]  KbParamMax=[]  KtParamMin=[]  KtParamMax=[]  KbOutMin=[]  KbOutMax=[]  KtOutMin=[]  KtOutMax=[]  IntegratorOutMin=[]  IntegratorOutMax=[]  FilterOutMin=[]  FilterOutMax=[]  SumI1OutMin=[]  SumI1OutMax=[]  SumI2OutMin=[]  SumI2OutMax=[]  SumI3OutMin=[]  SumI3OutMax=[]  SumI4OutMin=[]  SumI4OutMax=[]  SumDOutMin=[]  SumDOutMax=[]  DifferentiatorOutMin=[]  DifferentiatorOutMax=[]  FilterDiffOutCoefMin=[]  FilterDiffOutCoefMax=[]  ReciprocalOutMin=[]  ReciprocalOutMax=[]  SumDenOutMin=[]  SumDenOutMax=[]  SumNumOutMin=[]  SumNumOutMax=[]  DivideOutMin=[]  DivideOutMax=[]  UdiffTsProdOutMin=[]  UdiffTsProdOutMax=[]  NTsProdOutMin=[]  NTsProdOutMax=[]  UintegralTsProdOutMin=[]  UintegralTsProdOutMax=[]  UngainTsProdOutMin=[]  UngainTsProdOutMax=[]  ClampingZeroOutDataTypeStr=Inherit: Inherit via back propagation  ClampingZeroOutMin=[]  ClampingZeroOutMax=[]  FilterDenConstantOutDataTypeStr=Inherit: Inherit via back propagation  FilterDenConstantOutMin=[]  FilterDenConstantOutMax=[]  PCopyOutDataTypeStr=Inherit: Inherit via back propagation  PCopyOutMin=[]  PCopyOutMax=[]  NCopyOutDataTypeStr=Inherit: Inherit via back propagation  NCopyOutMin=[]  NCopyOutMax=[]  IntegratorContinuousStateAttributes=''  IntegratorStateMustResolveToSignalObject=off  IntegratorRTWStateStorageClass=Auto  FilterContinuousStateAttributes=''  FilterStateMustResolveToSignalObject=off  FilterRTWStateStorageClass=Auto  ParallelPVariant=InternalParameters  IdealPVariant=Disabled  IVariant=InternalParameters  DVariant=InternalParameters  IntegratorVariant=Continuous  SatVariant=Enabled  AWVariant=Passthrough  PCopyVariant=Disabled  TRVariant=Disabled  FdbkBlocksVariant=Forward  IdealPFdbkVariant=Disabled  SatFdbkVariant=Disabled  DerivativeFilterVariant=ContFilter  NVariant=InternalParameters  NCopyVariant=Disabled  FilterICVariant=InternalICsFilter  IntegratorICVariant=InternalICs  ExternalResetVariant=Disabled  TRSumVariant=Passthrough  SumFdbkVariant=Disabled  SumVariant=Sum_PID  TsampFilterVariant=InternalTs  TsampNgainVariant=Passthrough  TsampIntegralVariant=Disabled_SignalSpec  ExternalSaturationOutDataTypeStr=Inherit: Same as second input  DerivativeSourceVariant=ErrorSignal
  Constant : Constant  Value=I_z/I_z
  Constant1 : Constant  Value=K_psi_D1
  Constant2 : Constant  Value=psi_d
  Constant4 : Constant  Value=K_psi_P1
  Constant5 : Constant  Value=psi_d
  Derivative : Derivative
  Product : Product
  Product1 : Product
  Product2 : Product
  Sum : Sum  Inputs=++|
  Sum1 : Sum  Inputs=|+-
  Sum2 : Sum  Inputs=|+-
  tau_psi : Outport
  wires:
  Product/1 -> Sum/1
  Constant1/1 -> Product/1
  Product1/1 -> Sum/2
  Sum1/1 -> Product/2
  Constant4/1 -> Product1/1
  psi/1 -> Sum2/2
  Constant5/1 -> Sum2/1
  Derivative/1 -> Sum1/1
  Constant2/1 -> Derivative/1
  (psi)'/1 -> Sum1/2
  Sum2/1 -> Altitude controller/1, Product1/2
  Product2/1 -> tau_psi/1  "tau_psi"
  Constant/1 -> Product2/2
  Altitude controller/1 -> Product2/1
